simulink model "PMmotorFocECE517"  (R2018a)
settings: Solver=ode23t  StartTime=0  StopTime=0.1  FixedStep=1e-6  MaxStep=10e-7  RelTol=1e-8  EnableMultiTasking=on
InitFcn:
  | clc
  | clear
  | 
  | % DC Bus votlage
  | battery.Udc = 240;
  | 
  | % Motor
  | mtr.Ld = 400e-6;
  | mtr.Lq = 800e-6;
  | mtr.Rs = 0.05;
  | mtr.Lamda = 0.08;
  | mtr.Np = 3;
  | mtr.Jrotor = 0.03;
  | mtr.Tf = 3;
  | mtr.maxCurrLim = 280;
  | 
  | % inverter
  | Inv.RSnubber = 1e5;
  | Inv.Ron = 1e-3;
  | Inv.FrePWM = 10e3;
  | 
  | % current regulator
  | currCtrl.PI.wc = Inv.FrePWM/10*2*pi;
  | currCtrl.PI.Kpd = mtr.Ld*currCtrl.PI.wc;
  | currCtrl.PI.Kid = mtr.Rs*currCtrl.PI.wc;
  | currCtrl.PI.Kcd = 0.08;
  | currCtrl.PI.Kpq = mtr.Lq*currCtrl.PI.wc;
  | currCtrl.PI.Kiq = mtr.Rs*currCtrl.PI.wc;
  | currCtrl.PI.Kcq = 0.08;
  | currCtrl.voltageLim = battery.Udc*0.9;
  | 
  | % speed regulator
  | spdCtrl.PI.Kp = 12;
  | spdCtrl.PI.Ki= 3;
  | spdCtrl.PI.Kc  = 0.08;
  | 
  | %Field Weakening
  | fieldWeakening.PI.Kp = 0.3;
  | fieldWeakening.PI.Ki = 120;
  | fieldWeakening.PI.Kc = 3;
  | fieldWeakening.betaFLim = 90;  % deg
libraries: simulink x5, powerlib x5
settings Model: Creator=Rui Guan  LastModifiedBy=future
settings SolverCC: ZeroCrossControl=DisableAll  AlgebraicLoopSolver=LineSearch
settings DataIOCC: SaveFormat=Array  SignalLoggingSaveFormat=ModelDataLogs  SaveOutput=off  SignalLogging=off  DSMLogging=off  SaveTime=off
settings OptimizationCC: ExpressionDepthLimit=2147483647  LifeSpan=inf
settings DebuggingCC: UnderspecifiedInitializationDetection=Classic  MergeDetectMultiDrivingBlocksExec=none  SolverPrmCheckMsg=warning  FcnCallInpInsideContextMsg=warning  StateNameClashWarn=warning  SFUnexpectedBacktrackingDiag=warning  SFNoUnconditionalDefaultTransitionDiag=warning  SFExecutionAtInitializationDiag=none
settings HardwareCC: ProdBitPerPointer=32  ProdBitPerSizeT=32  ProdBitPerPtrDiffT=32  ProdLargestAtomicFloat=None  ProdIntDivRoundTo=Undefined  ProdEndianess=Unspecified  ProdWordSize=32  ProdHWDeviceType=32-bit Generic
settings ModelReferenceCC: PropagateSignalLabelsOutOfModel=off
settings CodeAppCC: StateflowObjectComments=on
settings GRTTargetCC: TargetLangStandard=C89/C90 (ANSI)  GeneratePreprocessorConditionals=Disable all  CombineOutputUpdateFcns=off  GRTInterface=on
settings ConfigComp: CovMetricSettings=dw  CovHtmlReporting=on  CovSaveCumulativeToWorkspaceVar=on  CovSaveSingleToWorkspaceVar=on  CovExternalEMLEnable=off
settings SimscapeCC: SimscapeNormalizeSystem=off

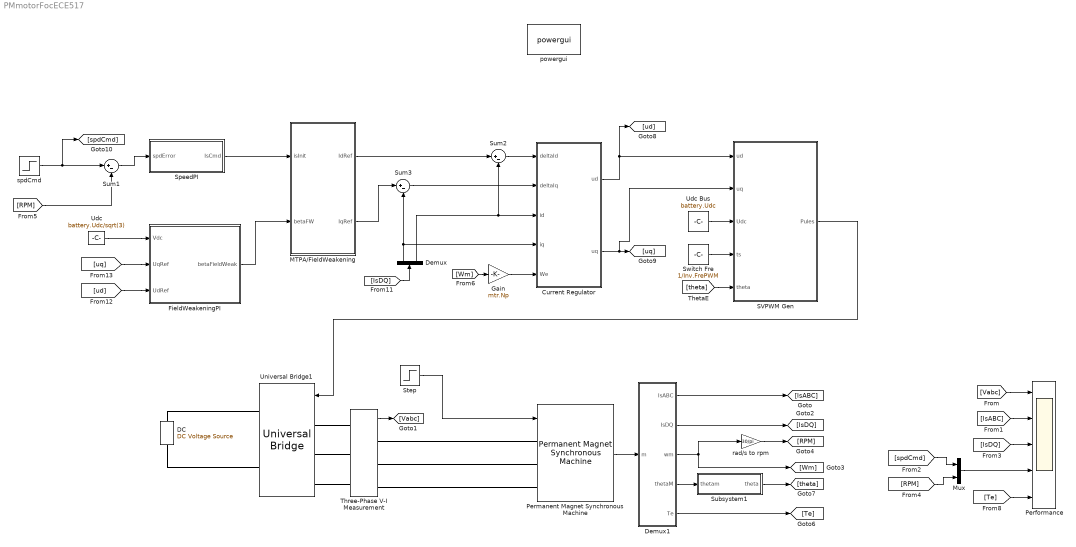
== system PMmotorFocECE517 ==
  " Udc Bus" : Constant  Value=battery.Udc
  " rad/s to rpm" : Gain  Gain=30/pi
  Current Regulator : Subsystem
  DC : powerlib/Electrical Sources/DC Voltage Source  Amplitude=battery.Udc  Measurements=Voltage
  Demux : Demux  Outputs=2
  Demux1 : Subsystem
  FieldWeakeningPI : Subsystem
  Gain : Gain  Gain=mtr.Np
  MTPA/FieldWeakening : Subsystem
  Mux : Mux  Inputs=2
  Performance : Scope  NumInputPorts=5
  Permanent Magnet Synchronous Machine : powerlib/Machines/Permanent Magnet Synchronous Machine  NbPhases=3  FluxDistribution=Sinusoidal  RotorType=Salient-pole  MechanicalLoad=Torque Tm  PresetModel=No  ShowDetailedParameters=on  MeasurementBus=off  Resistance=mtr.Rs  Inductance=8.5e-3  dqInductances=[mtr.Ld, mtr.Lq]  La=0.000835  MachineConstant=Flux linkage established by magnets (V.s)  Flux=mtr.Lamda  VoltageCst=43.5312  TorqueCst=0.36  Flat=120  Mechanical=[mtr.Jrotor 0 mtr.Tf]  PolePairs=3  InitialConditions=[0,0, 0,0]  InitialConditions5ph=[0 0 0 0 0 0]  TsPowergui=0  TsBlock=-1  RefAngle=90 degrees behind phase A axis (modified Park)
      settings: SourceProductName=Simscape Power Systems
  SVPWM Gen : Subsystem
  SpeedPI : Subsystem
  Step : Step  Time=0.2  Before=10  After=10  SampleTime=0
  Subsystem1 : Subsystem
  Sum1 : Sum  Inputs=|+-
  Sum2 : Sum  Inputs=|+-
  Sum3 : Sum  Inputs=|+-
  Switch Fre : Constant  Value=1/Inv.FrePWM  VectorParams1D=off
  Three-Phase V-I Measurement : powerlib/Measurements/Three-Phase V-I Measurement  VoltageMeasurement=phase-to-phase  SetLabelV=off  LabelV=Vabc  Vpu=off  VpuLL=off  CurrentMeasurement=no  SetLabelI=off  LabelI=Iabc  Ipu=off  Pbase=100e6  Vbase=500e3  OutputType=Complex  PhasorSimulation=off  PSBequivalent=0
  Udc : Constant  Value=battery.Udc/sqrt(3)
  Universal Bridge1 : powerlib/Power Electronics/Universal Bridge  Arms=3  SnubberResistance=Inv.RSnubber  SnubberCapacitance=inf  Device=IGBT / Diodes  Ron=Inv.Ron  Lon=0  ForwardVoltages="[  0  0  ]"  ForwardVoltage=0  GTOparameters=[ 10e-6 , 20e-6 ]  IGBTparameters=[ 1e-6 , 2e-6 ]  Measurements=None  Measurements_2=None  converterType=Rectifier
  powergui : powerlib/powergui  Priority=2  SimulationMode=Continuous  SampleTime=1e-6  frequency=60  Iterations=50  frequencyindice=0  Pbase=100e6  ErrMax=1e-4  UnitsV=kV  UnitsW=MW  buscounter=0  FunctionMessages=off  echomessages=off  EnableUseOfTLC=off  CurrentSourceSwitches=off  DisableSnubberDevices=off  DisableRonSwitches=off  DisableVfSwitches=off  DisplayEquations=off  SolverType=Tustin  Interpol=off  ExternalGateDelay=off  methode=off  Ts=0  x0status=blocks  SPID=off  SwTol=0  HookPort=off  RestoreLinks=warning  ResistiveCurrentMeasurement=off  Frange=[0:2:500]  Ylog=off  Xlog=on  ShowGrid=off  save=off  variable=ZData  structure=0  ZoomFFT=on  StartTime=0.0  cycles=1  DisplayStyle=1  fundamental=60  FreqAxis=off  MaxFrequency=1000  frequencyindicesteady=1  RmsSteady=1  display=off
  spdCmd : Step  Time=0.05  Before=1500  After=3000
  wires:
  Switch Fre/1 -> SVPWM Gen/4(ts)
  Permanent Magnet Synchronous Machine/1 -> Demux1/1(m)
  spdCmd/1 -> [spdCmd], Sum1/1
  Demux1/3(wm) -> " rad/s to rpm"/1, [Wm]
  Step/1 -> Permanent Magnet Synchronous Machine/1
  " Udc Bus"/1 -> SVPWM Gen/3(Udc)
  Sum2/1 -> Current Regulator/1(deltaId)
  Sum3/1 -> Current Regulator/2(deltaIq)
  MTPA/FieldWeakening/1(IdRef) -> Sum2/1
  MTPA/FieldWeakening/2(IqRef) -> Sum3/1
  SVPWM Gen/1(Pules) -> Universal Bridge1/1
  Three-Phase V-I Measurement/1 -> [Vabc]
  [Vabc] -> Performance/1
  Demux1/1(IsABC) -> [IsABC]
  [IsABC] -> Performance/2
  Demux1/2(IsDQ) -> [IsDQ]
  [IsDQ] -> Performance/3
  " rad/s to rpm"/1 -> [RPM]
  [RPM] -> Sum1/2
  [Wm] -> Gain/1
  Gain/1 -> Current Regulator/5(We)
  Demux1/4(thetaM) -> Subsystem1/1(thetam)
  Demux1/5(Te) -> [Te]
  [Te] -> Performance/5
  Subsystem1/1(theta) -> [theta]
  Demux/2 -> Sum2/2, Current Regulator/3(id)
  Demux/1 -> Sum3/2, Current Regulator/4(iq)
  [IsDQ] -> Demux/1
  Current Regulator/1(ud) -> [ud], SVPWM Gen/1(ud)
  Current Regulator/2(uq) -> SVPWM Gen/2(uq), [uq]
  FieldWeakeningPI/1(betaFieldWeak) -> MTPA/FieldWeakening/2(betaFW)
  Udc/1 -> FieldWeakeningPI/1(Vdc)
  [uq] -> FieldWeakeningPI/2(UqRef)
  [ud] -> FieldWeakeningPI/3(UdRef)
  Mux/1 -> Performance/4
  [RPM] -> Mux/2
  [spdCmd] -> Mux/1
  [theta] -> SVPWM Gen/5(theta)
  SpeedPI/1(IsCmd) -> MTPA/FieldWeakening/1(isInit)
  Sum1/1 -> SpeedPI/1(spdError)
  connections:
  DC/RConn1 -- Universal Bridge1/RConn1
  DC/LConn1 -- Universal Bridge1/RConn2
  Three-Phase V-I Measurement/LConn1 -- Universal Bridge1/LConn1
  Three-Phase V-I Measurement/LConn2 -- Universal Bridge1/LConn2
  Three-Phase V-I Measurement/LConn3 -- Universal Bridge1/LConn3
  Three-Phase V-I Measurement/RConn1 -- Permanent Magnet Synchronous Machine/LConn1
  Three-Phase V-I Measurement/RConn2 -- Permanent Magnet Synchronous Machine/LConn2
  Three-Phase V-I Measurement/RConn3 -- Permanent Magnet Synchronous Machine/LConn3

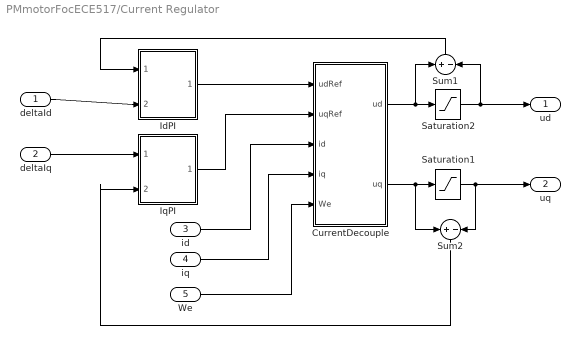
== system PMmotorFocECE517/Current Regulator ==
  deltaId : Inport
  deltaIq : Inport  Port=2
  id : Inport  Port=3
  iq : Inport  Port=4
  We : Inport  Port=5
  CurrentDecouple : Subsystem
  IdPI : Subsystem
  IqPI : Subsystem
  Saturation1 : Saturate  UpperLimit=currCtrl.voltageLim  LowerLimit=-currCtrl.voltageLim
  Saturation2 : Saturate  UpperLimit=currCtrl.voltageLim  LowerLimit=-currCtrl.voltageLim
  Sum1 : Sum  Inputs=+-  OutDataTypeStr=Inherit: Same as first input
  Sum2 : Sum  Inputs=+-  OutDataTypeStr=Inherit: Same as first input
  ud : Outport
  uq : Outport  Port=2
  wires:
  id/1 -> CurrentDecouple/3(id)
  CurrentDecouple/1(ud) -> Saturation2/1, Sum1/1
  iq/1 -> CurrentDecouple/4(iq)
  deltaIq/1 -> IqPI/1(iqError)
  IqPI/1(uqRef) -> CurrentDecouple/2(uqRef)
  We/1 -> CurrentDecouple/5(We)
  IdPI/1(udRef) -> CurrentDecouple/1(udRef)
  Saturation1/1 -> uq/1, Sum2/2
  CurrentDecouple/2(uq) -> Saturation1/1, Sum2/1
  Saturation2/1 -> ud/1, Sum1/2
  deltaId/1 -> IdPI/2(idError)
  Sum1/1 -> IdPI/1(udError)
  Sum2/1 -> IqPI/2(uqError)

== system PMmotorFocECE517/Demux1 ==
  m : Inport
  Bus Selector1 : BusSelector  OutputSignals=Stator current is_a (A),Stator current is_b (A),Stator current is_c (A),Stator current is_q (A),Stator current is_d (A),Rotor speed wm (rad/s),Rotor angle thetam (rad),Electromagnetic torque Te (N*m)
  Mux : Mux  Inputs=3
  Mux1 : Mux  Inputs=2
  IsABC : Outport
  IsDQ : Outport  Port=2
  wm : Outport  Port=3
  thetaM : Outport  Port=4
  Te : Outport  Port=5
  wires:
  m/1 -> Bus Selector1/1
  Bus Selector1/1 -> Mux/1  "<Stator current is_a (A)>"
  Bus Selector1/2 -> Mux/2  "<Stator current is_b (A)>"
  Bus Selector1/3 -> Mux/3  "<Stator current is_c (A)>"
  Bus Selector1/6 -> wm/1  "<Rotor speed wm (rad/s)>"
  Bus Selector1/7 -> thetaM/1  "<Rotor angle thetam (rad)>"
  Bus Selector1/8 -> Te/1  "<Electromagnetic torque Te (N*m)>"
  Mux/1 -> IsABC/1
  Bus Selector1/5 -> Mux1/2  "<Stator current is_d (A)>"
  Bus Selector1/4 -> Mux1/1  "<Stator current is_q (A)>"
  Mux1/1 -> IsDQ/1

== system PMmotorFocECE517/FieldWeakeningPI ==
  Vdc : Inport
  UqRef : Inport  Port=2
  UdRef : Inport  Port=3
  FieldWeakeningPICtrl : Subsystem
  Mux2 : Mux  Inputs=2
  Saturation : Saturate  UpperLimit=0  LowerLimit=-fieldWeakening.betaFLim
  Sum4 : Sum  Inputs=+-
  UMag : Fcn  Expr=sqrt(u[1]^2+u[2]^2)
  betaFieldWeak : Outport
  wires:
  UqRef/1 -> Mux2/1
  UdRef/1 -> Mux2/2
  Sum4/1 -> FieldWeakeningPICtrl/1(Error)
  Saturation/1 -> betaFieldWeak/1
  Vdc/1 -> Sum4/1
  UMag/1 -> Sum4/2
  Mux2/1 -> UMag/1
  FieldWeakeningPICtrl/1(Betaf) -> Saturation/1

== system PMmotorFocECE517/MTPA//FieldWeakening ==
  isInit : Inport
  betaFW : Inport  Port=2
  CurrentBetaToIdIq : Subsystem
  MTPA : Subsystem
  Sum5 : Sum  Inputs=+-
  IdRef : Outport
  IqRef : Outport  Port=2
  wires:
  MTPA/1(beta) -> Sum5/1
  isInit/1 -> MTPA/1(is), CurrentBetaToIdIq/2(is)
  betaFW/1 -> Sum5/2
  CurrentBetaToIdIq/1(id) -> IdRef/1
  CurrentBetaToIdIq/2(iq) -> IqRef/1
  Sum5/1 -> CurrentBetaToIdIq/1("beta ")

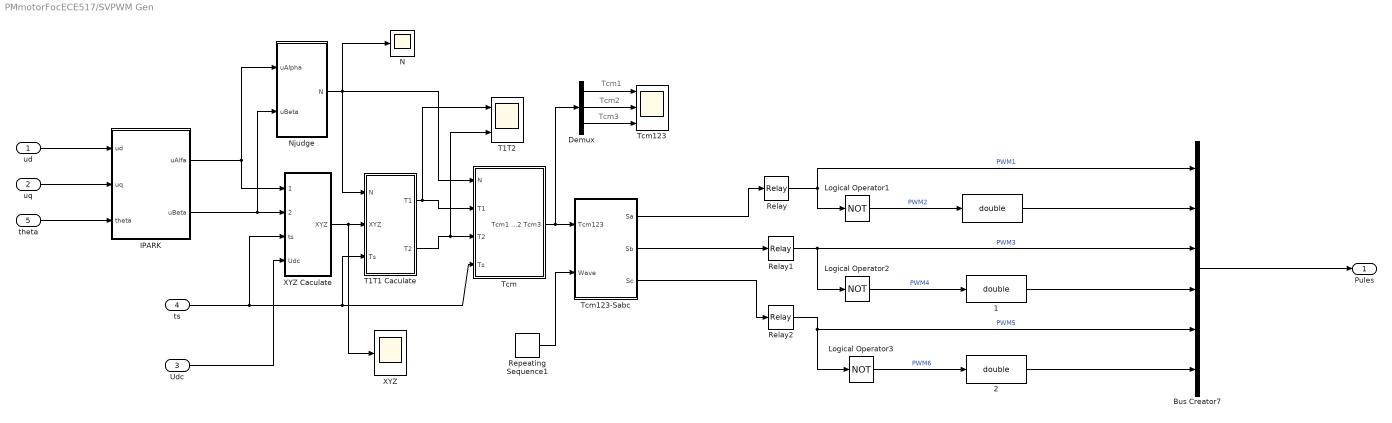
== system PMmotorFocECE517/SVPWM Gen ==
  note: Tcm1
  note: Tcm2
  note: Tcm3
  ud : Inport
  uq : Inport  Port=2
  Udc : Inport  Port=3
  ts : Inport  Port=4
  theta : Inport  Port=5
  "  " : DataTypeConversion  OutDataTypeStr=double
  "  1" : DataTypeConversion  OutDataTypeStr=double
  "  2" : DataTypeConversion  OutDataTypeStr=double
  Bus Creator7 : BusCreator  Inputs=6
  Demux : Demux  Outputs=3
  "IPARK " : Subsystem
  Logical Operator1 : Logic  Operator=NOT  AllPortsSameDT=off
  Logical Operator2 : Logic  Operator=NOT  AllPortsSameDT=off
  Logical Operator3 : Logic  Operator=NOT  AllPortsSameDT=off
  N : Scope
  Njudge : Subsystem
  Relay : Relay
  Relay1 : Relay
  Relay2 : Relay
  Repeating Sequence1 : simulink/Sources/Repeating Sequence  rep_seq_t="[0 1/2/Inv.FrePWM  1/Inv.FrePWM]"  rep_seq_y=[0 1/2/Inv.FrePWM 0]
  T1T1 Caculate : Subsystem  TreatAsAtomicUnit=on
  T1T2 : Scope  NumInputPorts=2
  Tcm : Subsystem
  Tcm123 : Scope  NumInputPorts=3
  Tcm123-Sabc : Subsystem
  XYZ : Scope
  "XYZ Caculate " : Subsystem
  Pules : Outport
  wires:
  "IPARK "/1(uAlfa) -> "XYZ Caculate "/1(uAlpha), Njudge/1(uAlpha)
  "XYZ Caculate "/1(XYZ) -> XYZ/1, T1T1 Caculate/2(XYZ)
  T1T1 Caculate/1(T1) -> T1T2/1, Tcm/2(T1)
  T1T1 Caculate/2(T2) -> T1T2/2, Tcm/3(T2)
  Njudge/1("N ") -> N/1, T1T1 Caculate/1(N), Tcm/1(N)
  Tcm/1(Tcm1 Tcm2 Tcm3) -> Demux/1, Tcm123-Sabc/1(Tcm123)
  Repeating Sequence1/1 -> Tcm123-Sabc/2(Wave)
  Demux/1 -> Tcm123/1
  Demux/2 -> Tcm123/2
  Demux/3 -> Tcm123/3
  Udc/1 -> "XYZ Caculate "/4(Udc)
  ts/1 -> "XYZ Caculate "/3(ts), T1T1 Caculate/3(Ts), Tcm/4(Ts)
  "IPARK "/2(uBeta) -> "XYZ Caculate "/2(uBeta), Njudge/2(uBeta)
  "  2"/1 -> Bus Creator7/6
  Logical Operator3/1 -> "  2"/1  "PWM6"
  "  1"/1 -> Bus Creator7/4
  Logical Operator2/1 -> "  1"/1  "PWM4"
  Logical Operator1/1 -> "  "/1  "PWM2"
  "  "/1 -> Bus Creator7/2
  Bus Creator7/1 -> Pules/1
  Relay2/1 -> Bus Creator7/5, Logical Operator3/1  "PWM5"
  Relay1/1 -> Bus Creator7/3, Logical Operator2/1  "PWM3"
  Relay/1 -> Bus Creator7/1, Logical Operator1/1  "PWM1"
  Tcm123-Sabc/3(Sc) -> Relay2/1
  Tcm123-Sabc/2(Sb) -> Relay1/1
  Tcm123-Sabc/1(Sa) -> Relay/1
  ud/1 -> "IPARK "/1(ud)
  uq/1 -> "IPARK "/2(uq)
  theta/1 -> "IPARK "/3(theta)

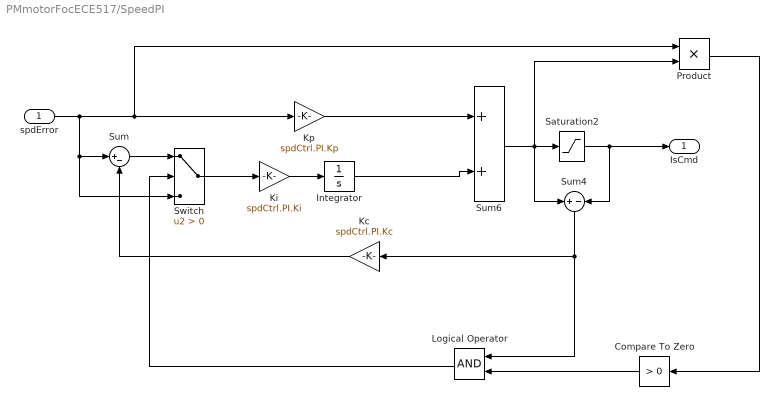
== system PMmotorFocECE517/SpeedPI ==
  spdError : Inport
  Compare To Zero : simulink/Logic and Bit Operations/Compare To Zero  relop=>  OutDataTypeStr=uint8  ZeroCross=off
  Integrator : Integrator
  Kc : Gain  Gain=spdCtrl.PI.Kc  OutDataTypeStr=Inherit: Same as input  ParamDataTypeStr=Inherit: Same as input
  Ki : Gain  Gain=spdCtrl.PI.Ki  OutDataTypeStr=Inherit: Same as input  ParamDataTypeStr=Inherit: Same as input
  Kp : Gain  Gain=spdCtrl.PI.Kp  OutDataTypeStr=Inherit: Same as input  ParamDataTypeStr=Inherit: Same as input
  Logical Operator : Logic  AllPortsSameDT=off  OutDataTypeStr=boolean
  Product : Product  RndMeth=Zero
  Saturation2 : Saturate  UpperLimit=mtr.maxCurrLim  LowerLimit=-mtr.maxCurrLim
  Sum : Sum  Inputs=|+-  OutDataTypeStr=Inherit: Same as first input
  Sum4 : Sum  Inputs=+-  OutDataTypeStr=Inherit: Same as first input
  Sum6 : Sum  SaturateOnIntegerOverflow=on  InputSameDT=on  OutDataTypeStr=Inherit: Same as first input
  Switch : Switch  Criteria=u2 > Threshold
  IsCmd : Outport
  wires:
  Compare To Zero/1 -> Logical Operator/2
  Sum4/1 -> Logical Operator/1, Kc/1
  Sum6/1 -> Saturation2/1, Sum4/1, Product/2
  Sum/1 -> Switch/1
  Product/1 -> Compare To Zero/1
  Logical Operator/1 -> Switch/2
  Switch/1 -> Ki/1
  Ki/1 -> Integrator/1
  Integrator/1 -> Sum6/2
  Saturation2/1 -> IsCmd/1, Sum4/2
  Kc/1 -> Sum/2
  Kp/1 -> Sum6/1
  spdError/1 -> Kp/1, Product/1, Sum/1, Switch/3

== system PMmotorFocECE517/Subsystem1 ==
  thetam : Inport
  Add1 : Sum  Inputs=+-
  Constant4 : Constant  Value=0.5*pi
  Gain1 : Gain  Gain=mtr.Np
  theta : Outport
  wires:
  Gain1/1 -> Add1/1
  Constant4/1 -> Add1/2
  Add1/1 -> theta/1
  thetam/1 -> Gain1/1

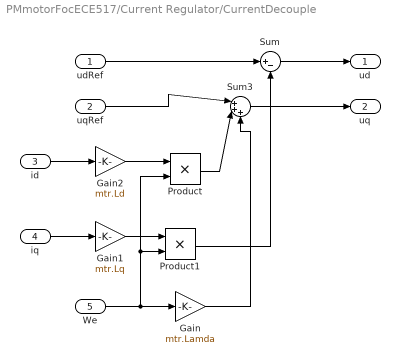
== system PMmotorFocECE517/Current Regulator/CurrentDecouple ==
  udRef : Inport
  uqRef : Inport  Port=2
  id : Inport  Port=3
  iq : Inport  Port=4
  We : Inport  Port=5
  Gain : Gain  Gain=mtr.Lamda
  Gain1 : Gain  Gain=mtr.Lq
  Gain2 : Gain  Gain=mtr.Ld
  Product : Product  RndMeth=Zero
  Product1 : Product  RndMeth=Zero
  Sum : Sum  Inputs=|+-
  Sum3 : Sum  Inputs=|+++
  ud : Outport
  uq : Outport  Port=2
  wires:
  Sum3/1 -> uq/1
  Product/1 -> Sum3/2
  uqRef/1 -> Sum3/1
  Gain/1 -> Sum3/3
  We/1 -> Product/2, Product1/2, Gain/1
  iq/1 -> Gain1/1
  udRef/1 -> Sum/1
  Product1/1 -> Sum/2
  Sum/1 -> ud/1
  Gain1/1 -> Product1/1
  Gain2/1 -> Product/1
  id/1 -> Gain2/1

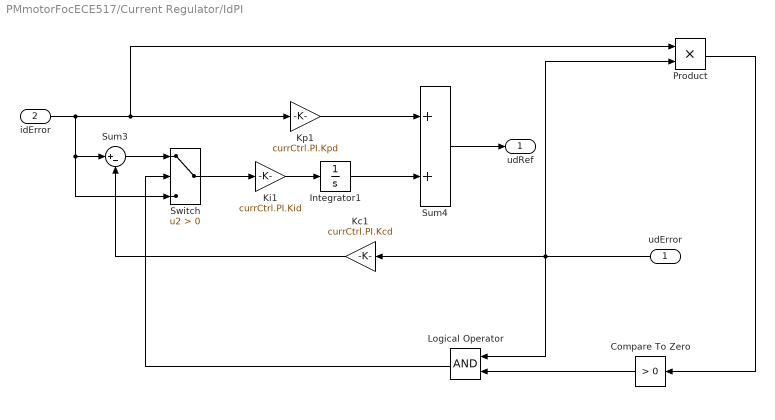
== system PMmotorFocECE517/Current Regulator/IdPI ==
  udError : Inport
  idError : Inport  Port=2
  Compare To Zero : simulink/Logic and Bit Operations/Compare To Zero  relop=>  OutDataTypeStr=uint8  ZeroCross=off
  Integrator1 : Integrator
  Kc1 : Gain  Gain=currCtrl.PI.Kcd  OutDataTypeStr=Inherit: Same as input  ParamDataTypeStr=Inherit: Same as input
  Ki1 : Gain  Gain=currCtrl.PI.Kid  OutDataTypeStr=Inherit: Same as input  ParamDataTypeStr=Inherit: Same as input
  Kp1 : Gain  Gain=currCtrl.PI.Kpd  OutDataTypeStr=Inherit: Same as input  ParamDataTypeStr=Inherit: Same as input
  Logical Operator : Logic  AllPortsSameDT=off  OutDataTypeStr=boolean
  Product : Product  RndMeth=Zero
  Sum3 : Sum  Inputs=|+-  OutDataTypeStr=Inherit: Same as first input
  Sum4 : Sum  SaturateOnIntegerOverflow=on  InputSameDT=on  OutDataTypeStr=Inherit: Same as first input
  Switch : Switch  Criteria=u2 > Threshold
  udRef : Outport
  wires:
  Switch/1 -> Ki1/1
  Ki1/1 -> Integrator1/1
  Sum4/1 -> udRef/1
  udError/1 -> Kc1/1, Product/2, Logical Operator/1
  Integrator1/1 -> Sum4/2
  Sum3/1 -> Switch/1
  Kc1/1 -> Sum3/2
  Kp1/1 -> Sum4/1
  Compare To Zero/1 -> Logical Operator/2
  Logical Operator/1 -> Switch/2
  idError/1 -> Kp1/1, Product/1, Sum3/1, Switch/3
  Product/1 -> Compare To Zero/1

== system PMmotorFocECE517/Current Regulator/IqPI ==
  iqError : Inport
  uqError : Inport  Port=2
  Compare To Zero : simulink/Logic and Bit Operations/Compare To Zero  relop=>  OutDataTypeStr=uint8  ZeroCross=off
  Integrator1 : Integrator
  Kc1 : Gain  Gain=currCtrl.PI.Kcq  OutDataTypeStr=Inherit: Same as input  ParamDataTypeStr=Inherit: Same as input
  Ki1 : Gain  Gain=currCtrl.PI.Kiq  OutDataTypeStr=Inherit: Same as input  ParamDataTypeStr=Inherit: Same as input
  Kp1 : Gain  Gain=currCtrl.PI.Kpq  OutDataTypeStr=Inherit: Same as input  ParamDataTypeStr=Inherit: Same as input
  Logical Operator : Logic  AllPortsSameDT=off  OutDataTypeStr=boolean
  Product : Product  RndMeth=Zero
  Sum3 : Sum  Inputs=|+-  OutDataTypeStr=Inherit: Same as first input
  Sum4 : Sum  SaturateOnIntegerOverflow=on  InputSameDT=on  OutDataTypeStr=Inherit: Same as first input
  Switch : Switch  Criteria=u2 > Threshold
  uqRef : Outport
  wires:
  Ki1/1 -> Integrator1/1
  Integrator1/1 -> Sum4/2
  Product/1 -> Compare To Zero/1
  Switch/1 -> Ki1/1
  iqError/1 -> Kp1/1, Product/1, Sum3/1, Switch/3
  Compare To Zero/1 -> Logical Operator/2
  Logical Operator/1 -> Switch/2
  Kp1/1 -> Sum4/1
  Sum3/1 -> Switch/1
  Sum4/1 -> uqRef/1
  uqError/1 -> Kc1/1, Product/2, Logical Operator/1
  Kc1/1 -> Sum3/2

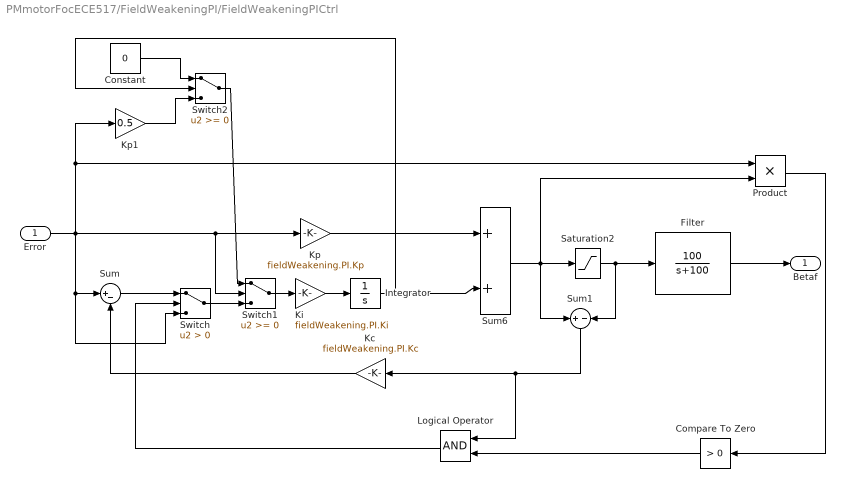
== system PMmotorFocECE517/FieldWeakeningPI/FieldWeakeningPICtrl ==
  Error : Inport
  Compare To Zero : simulink/Logic and Bit Operations/Compare To Zero  relop=>  OutDataTypeStr=uint8  ZeroCross=off
  Constant : Constant  Value=0
  Filter : TransferFcn  Numerator=[100]  Denominator=[1 100]
  Integrator : Integrator
  Kc : Gain  Gain=fieldWeakening.PI.Kc  OutDataTypeStr=Inherit: Same as input  ParamDataTypeStr=Inherit: Same as input
  Ki : Gain  Gain=fieldWeakening.PI.Ki  OutDataTypeStr=Inherit: Same as input  ParamDataTypeStr=Inherit: Same as input
  Kp : Gain  Gain=fieldWeakening.PI.Kp  OutDataTypeStr=Inherit: Same as input  ParamDataTypeStr=Inherit: Same as input
  Kp1 : Gain  Gain=0.5  OutDataTypeStr=Inherit: Same as input  ParamDataTypeStr=Inherit: Same as input
  Logical Operator : Logic  AllPortsSameDT=off  OutDataTypeStr=boolean
  Product : Product  RndMeth=Zero
  Saturation2 : Saturate  UpperLimit=fieldWeakening.betaFLim  LowerLimit=-fieldWeakening.betaFLim
  Sum : Sum  Inputs=|+-  OutDataTypeStr=Inherit: Same as first input
  Sum1 : Sum  Inputs=+-  OutDataTypeStr=Inherit: Same as first input
  Sum6 : Sum  SaturateOnIntegerOverflow=on  InputSameDT=on  OutDataTypeStr=Inherit: Same as first input
  Switch : Switch  Criteria=u2 > Threshold
  Switch1 : Switch
  Switch2 : Switch
  Betaf : Outport
  wires:
  Kp/1 -> Sum6/1
  Switch1/1 -> Ki/1
  Kp1/1 -> Switch2/3
  Kc/1 -> Sum/2
  Constant/1 -> Switch2/1
  Product/1 -> Compare To Zero/1
  Sum1/1 -> Kc/1, Logical Operator/1
  Error/1 -> Kp/1, Switch1/2, Product/1, Kp1/1, Sum/1, Switch/3
  Switch/1 -> Switch1/3
  Ki/1 -> Integrator/1
  Integrator/1 -> Sum6/2, Switch2/2
  Sum/1 -> Switch/1
  Compare To Zero/1 -> Logical Operator/2
  Switch2/1 -> Switch1/1
  Logical Operator/1 -> Switch/2
  Filter/1 -> Betaf/1
  Sum6/1 -> Product/2, Sum1/1, Saturation2/1
  Saturation2/1 -> Filter/1, Sum1/2

== system PMmotorFocECE517/MTPA//FieldWeakening/CurrentBetaToIdIq ==
  "beta " : Inport
  is : Inport  Port=2
  Gain1 : Gain  Gain=pi/180
  Product : Product  RndMeth=Zero
  Product1 : Product  RndMeth=Zero
  Trigonometric Function : Trigonometry
  Trigonometric Function1 : Trigonometry  Operator=cos
  id : Outport
  iq : Outport  Port=2
  wires:
  Product/1 -> iq/1
  Product1/1 -> id/1
  Trigonometric Function/1 -> Product/1
  "beta "/1 -> Gain1/1
  is/1 -> Product1/1, Product/2
  Gain1/1 -> Trigonometric Function/1, Trigonometric Function1/1
  Trigonometric Function1/1 -> Product1/2

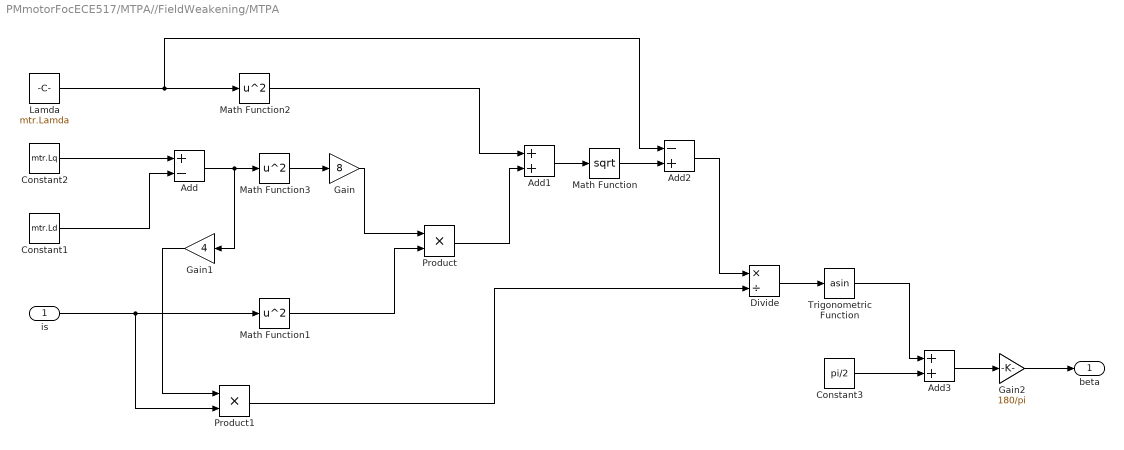
== system PMmotorFocECE517/MTPA//FieldWeakening/MTPA ==
  is : Inport
  Add : Sum  Inputs=+-
  Add1 : Sum
  Add2 : Sum  Inputs=-+
  Add3 : Sum
  Constant1 : Constant  Value=mtr.Ld
  Constant2 : Constant  Value=mtr.Lq
  Constant3 : Constant  Value=pi/2
  Divide : Product  Inputs=*/
  Gain : Gain  Gain=8
  Gain1 : Gain  Gain=4
  Gain2 : Gain  Gain=180/pi
  Lamda : Constant  Value=mtr.Lamda
  Math Function : Math  Operator=sqrt  SaturateOnIntegerOverflow=on
  Math Function1 : Math  Operator=square  SaturateOnIntegerOverflow=on
  Math Function2 : Math  Operator=square  SaturateOnIntegerOverflow=on
  Math Function3 : Math  Operator=square  SaturateOnIntegerOverflow=on
  Product : Product  RndMeth=Zero
  Product1 : Product  RndMeth=Zero
  Trigonometric Function : Trigonometry  Operator=asin
  beta : Outport
  wires:
  Divide/1 -> Trigonometric Function/1
  Add1/1 -> Math Function/1
  Math Function/1 -> Add2/2
  Gain2/1 -> beta/1
  Constant1/1 -> Add/2
  Trigonometric Function/1 -> Add3/1
  is/1 -> Product1/2, Math Function1/1
  Add3/1 -> Gain2/1
  Add/1 -> Math Function3/1, Gain1/1
  Gain/1 -> Product/1
  Math Function2/1 -> Add1/1
  Gain1/1 -> Product1/1
  Product/1 -> Add1/2
  Product1/1 -> Divide/2
  Math Function3/1 -> Gain/1
  Math Function1/1 -> Product/2
  Lamda/1 -> Math Function2/1, Add2/1
  Add2/1 -> Divide/1
  Constant2/1 -> Add/1
  Constant3/1 -> Add3/2

== system PMmotorFocECE517/SVPWM Gen/IPARK  ==
  ud : Inport
  uq : Inport  Port=2
  theta : Inport  Port=3
  Mux : Mux  Inputs=3
  uAlfaFuc : Fcn  Expr=u(1)*cos(u(3))-u(2)*sin(u(3))
  uBetaFuc : Fcn  Expr=u(1)*sin(u(3))+u(2)*cos(u(3))
  uAlfa : Outport
  uBeta : Outport  Port=2
  wires:
  uBetaFuc/1 -> uBeta/1
  theta/1 -> Mux/3
  uq/1 -> Mux/2
  ud/1 -> Mux/1
  uAlfaFuc/1 -> uAlfa/1
  Mux/1 -> uBetaFuc/1, uAlfaFuc/1

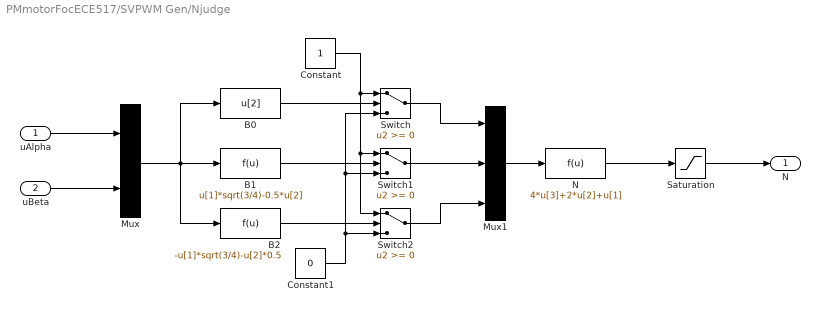
== system PMmotorFocECE517/SVPWM Gen/Njudge ==
  uAlpha : Inport
  uBeta : Inport  Port=2
  B0 : Fcn  Expr=u[2]
  B1 : Fcn  Expr=u[1]*sqrt(3/4)-0.5*u[2]
  B2 : Fcn  Expr=-u[1]*sqrt(3/4)-u[2]*0.5
  Constant : Constant
  Constant1 : Constant  Value=0
  Mux : Mux  Inputs=2
  Mux1 : Mux  Inputs=3
  N : Fcn  Expr=4*u[3]+2*u[2]+u[1]
  Saturation : Saturate  UpperLimit=6  LowerLimit=1
  Switch : Switch
  Switch1 : Switch
  Switch2 : Switch
  "N " : Outport
  wires:
  N/1 -> Saturation/1
  Mux1/1 -> N/1
  Switch1/1 -> Mux1/2
  Constant1/1 -> Switch2/3, Switch1/3, Switch/3
  Constant/1 -> Switch1/1, Switch2/1, Switch/1
  B2/1 -> Switch2/2
  B1/1 -> Switch1/2
  B0/1 -> Switch/2
  Mux/1 -> B2/1, B0/1, B1/1
  uBeta/1 -> Mux/2
  uAlpha/1 -> Mux/1
  Switch/1 -> Mux1/1
  Switch2/1 -> Mux1/3
  Saturation/1 -> "N "/1

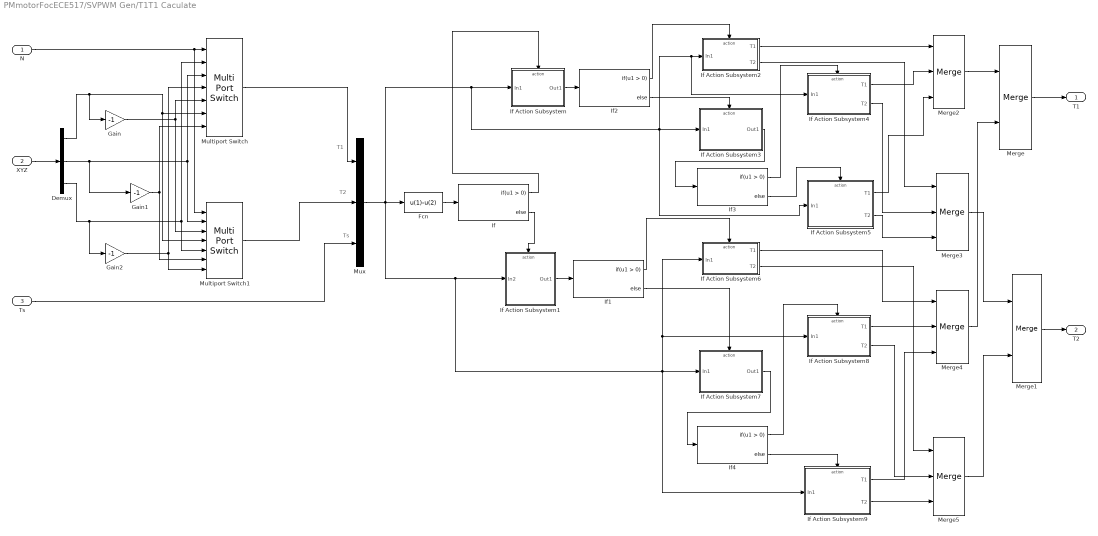
== system PMmotorFocECE517/SVPWM Gen/T1T1 Caculate ==
  note: Ts
  note: T2
  note: T1
  N : Inport
  XYZ : Inport  Port=2
  Ts : Inport  Port=3
  Demux : Demux  Outputs=3
  Fcn : Fcn  Expr=u(1)-u(2)
  Gain : Gain  Gain=-1  OutDataTypeStr=Inherit: Same as input  ParamDataTypeStr=Inherit: Same as input
  Gain1 : Gain  Gain=-1  OutDataTypeStr=Inherit: Same as input  ParamDataTypeStr=Inherit: Same as input
  Gain2 : Gain  Gain=-1  OutDataTypeStr=Inherit: Same as input  ParamDataTypeStr=Inherit: Same as input
  If{,1..4} (5 alike) : If
  If Action Subsystem : Subsystem  TreatAsAtomicUnit=on
  If Action Subsystem1 : Subsystem  TreatAsAtomicUnit=on
  If Action Subsystem2 : Subsystem  TreatAsAtomicUnit=on
  If Action Subsystem3 : Subsystem  TreatAsAtomicUnit=on
  If Action Subsystem4 : Subsystem  TreatAsAtomicUnit=on
  If Action Subsystem5 : Subsystem  TreatAsAtomicUnit=on
  If Action Subsystem6 : Subsystem  TreatAsAtomicUnit=on
  If Action Subsystem7 : Subsystem  TreatAsAtomicUnit=on
  If Action Subsystem8 : Subsystem  TreatAsAtomicUnit=on
  If Action Subsystem9 : Subsystem  TreatAsAtomicUnit=on
  Merge : Merge
  Merge1 : Merge
  Merge{2..5} (4 alike) : Merge  Inputs=3
  Multiport Switch : MultiPortSwitch  Inputs=6
  Multiport Switch1 : MultiPortSwitch  Inputs=6
  Mux : Mux  Inputs=3
  T1 : Outport
  T2 : Outport  Port=2
  wires:
  If4/2 -> If Action Subsystem9/Action
  If4/1 -> If Action Subsystem8/Action
  If Action Subsystem7/1(Out1) -> If4/1
  If3/2 -> If Action Subsystem5/Action
  If3/1 -> If Action Subsystem4/Action
  If Action Subsystem3/1(Out1) -> If3/1
  If1/1 -> If Action Subsystem6/Action
  If Action Subsystem1/1(Out1) -> If1/1
  If2/2 -> If Action Subsystem3/Action
  If2/1 -> If Action Subsystem2/Action
  If Action Subsystem/1(Out1) -> If2/1
  Gain1/1 -> Multiport Switch/7, Multiport Switch1/6
  Gain2/1 -> Multiport Switch1/7, Multiport Switch/4
  Gain/1 -> Multiport Switch/5, Multiport Switch1/3
  Demux/1 -> Gain/1, Multiport Switch1/4, Multiport Switch/6
  Demux/3 -> Gain2/1, Multiport Switch/2, Multiport Switch1/5
  Demux/2 -> Gain1/1, Multiport Switch1/2, Multiport Switch/3
  Multiport Switch1/1 -> Mux/2
  Multiport Switch/1 -> Mux/1
  Mux/1 -> If Action Subsystem9/1(In1), If Action Subsystem8/1(In1), If Action Subsystem6/1(In1), If Action Subsystem7/1(In1), If Action Subsystem1/1(In2), If Action Subsystem/1(In1), If Action Subsystem5/1(In1), If Action Subsystem4/1(In1), If Action Subsystem2/1(In1), If Action Subsystem3/1(In1), Fcn/1
  XYZ/1 -> Demux/1
  Ts/1 -> Mux/3
  Fcn/1 -> If/1
  If/1 -> If Action Subsystem/Action
  If/2 -> If Action Subsystem1/Action
  Merge/1 -> T1/1
  Merge1/1 -> T2/1
  If Action Subsystem8/1(T1) -> Merge4/2
  If1/2 -> If Action Subsystem7/Action
  If Action Subsystem2/1(T1) -> Merge2/1
  If Action Subsystem4/1(T1) -> Merge2/2
  If Action Subsystem5/1(T1) -> Merge2/3
  If Action Subsystem2/2(T2) -> Merge3/1
  If Action Subsystem4/2(T2) -> Merge3/2
  If Action Subsystem5/2(T2) -> Merge3/3
  Merge2/1 -> Merge/1
  Merge3/1 -> Merge1/1
  Merge4/1 -> Merge/2
  Merge5/1 -> Merge1/2
  If Action Subsystem6/1(T1) -> Merge4/1
  If Action Subsystem9/1(T1) -> Merge4/3
  If Action Subsystem6/2(T2) -> Merge5/1
  If Action Subsystem8/2(T2) -> Merge5/2
  If Action Subsystem9/2(T2) -> Merge5/3
  N/1 -> Multiport Switch1/1, Multiport Switch/1

== system PMmotorFocECE517/SVPWM Gen/Tcm ==
  N : Inport
  T1 : Inport  Port=2
  T2 : Inport  Port=3
  Ts : Inport  Port=4
  Fcn : Fcn  Expr=(u[3]-u[1]-u[2])/4
  Fcn1 : Fcn  Expr=(u[3]+u[1]-u[2])/4
  Fcn2 : Fcn  Expr=(u[3]+u[2]+u[1])/4
  Multiport Switch : MultiPortSwitch  Inputs=6
  Multiport Switch1 : MultiPortSwitch  Inputs=6
  Multiport Switch2 : MultiPortSwitch  Inputs=6
  Mux : Mux  Inputs=3
  Mux1 : Mux  Inputs=3
  Tcm1 Tcm2 Tcm3 : Outport
  wires:
  N/1 -> Multiport Switch2/1, Multiport Switch1/1, Multiport Switch/1
  Fcn2/1 -> Multiport Switch2/4, Multiport Switch2/2, Multiport Switch1/7, Multiport Switch1/3, Multiport Switch/6, Multiport Switch/5
  Fcn1/1 -> Multiport Switch2/6, Multiport Switch2/3, Multiport Switch1/5, Multiport Switch1/4, Multiport Switch/2, Multiport Switch/7
  Fcn/1 -> Multiport Switch2/7, Multiport Switch2/5, Multiport Switch1/6, Multiport Switch1/2, Multiport Switch/4, Multiport Switch/3
  Mux1/1 -> Tcm1 Tcm2 Tcm3/1
  Multiport Switch/1 -> Mux1/1
  Multiport Switch1/1 -> Mux1/2
  Multiport Switch2/1 -> Mux1/3
  T1/1 -> Mux/1
  T2/1 -> Mux/2
  Ts/1 -> Mux/3
  Mux/1 -> Fcn1/1, Fcn/1, Fcn2/1

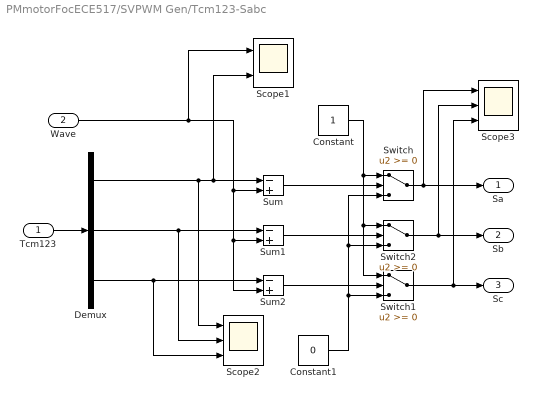
== system PMmotorFocECE517/SVPWM Gen/Tcm123-Sabc ==
  Tcm123 : Inport
  Wave : Inport  Port=2
  Constant : Constant
  Constant1 : Constant  Value=0
  Demux : Demux  Outputs=3
  Scope1 : Scope  NumInputPorts=2
  Scope2 : Scope  NumInputPorts=3
  Scope3 : Scope  NumInputPorts=3
  Sum : Sum  Inputs=-+  SaturateOnIntegerOverflow=on  OutDataTypeStr=Inherit: Same as first input
  Sum1 : Sum  Inputs=-+  SaturateOnIntegerOverflow=on  OutDataTypeStr=Inherit: Same as first input
  Sum2 : Sum  Inputs=-+  SaturateOnIntegerOverflow=on  OutDataTypeStr=Inherit: Same as first input
  Switch : Switch  SaturateOnIntegerOverflow=on
  Switch1 : Switch  SaturateOnIntegerOverflow=on
  Switch2 : Switch  SaturateOnIntegerOverflow=on
  Sa : Outport
  Sb : Outport  Port=2
  Sc : Outport  Port=3
  wires:
  Wave/1 -> Scope1/1, Sum/2, Sum2/2, Sum1/2
  Demux/1 -> Scope2/1, Sum/1, Scope1/2
  Demux/2 -> Scope2/2, Sum1/1
  Demux/3 -> Scope2/3, Sum2/1
  Tcm123/1 -> Demux/1
  Sum/1 -> Switch/2
  Sum1/1 -> Switch2/2
  Sum2/1 -> Switch1/2
  Constant/1 -> Switch1/1, Switch2/1, Switch/1
  Constant1/1 -> Switch/3, Switch2/3, Switch1/3
  Switch/1 -> Scope3/1, Sa/1
  Switch2/1 -> Scope3/2, Sb/1
  Switch1/1 -> Scope3/3, Sc/1

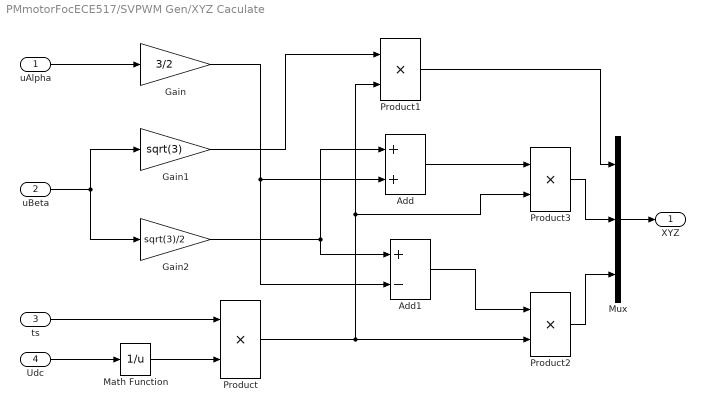
== system PMmotorFocECE517/SVPWM Gen/XYZ Caculate  ==
  uAlpha : Inport
  uBeta : Inport  Port=2
  ts : Inport  Port=3
  Udc : Inport  Port=4
  Add : Sum  OutDataTypeStr=Inherit: Same as first input
  Add1 : Sum  Inputs=+-  OutDataTypeStr=Inherit: Same as first input
  Gain : Gain  Gain=3/2  OutDataTypeStr=Inherit: Same as input  ParamDataTypeStr=Inherit: Same as input
  Gain1 : Gain  Gain=sqrt(3)  OutDataTypeStr=Inherit: Same as input  ParamDataTypeStr=Inherit: Same as input
  Gain2 : Gain  Gain=sqrt(3)/2  OutDataTypeStr=Inherit: Same as input  ParamDataTypeStr=Inherit: Same as input
  Math Function : Math  Operator=reciprocal  SaturateOnIntegerOverflow=on
  Mux : Mux  Inputs=3
  Product{,1..3} (4 alike) : Product  RndMeth=Zero  OutDataTypeStr=Inherit: Same as first input
  XYZ : Outport
  wires:
  Add/1 -> Product3/1
  Add1/1 -> Product2/1
  Gain2/1 -> Add1/1, Add/1
  Gain/1 -> Add/2, Add1/2
  Product/1 -> Product3/2, Product1/2, Product2/2
  Gain1/1 -> Product1/1
  ts/1 -> Product/1
  Math Function/1 -> Product/2
  Udc/1 -> Math Function/1
  uBeta/1 -> Gain1/1, Gain2/1
  uAlpha/1 -> Gain/1
  Product2/1 -> Mux/3
  Product3/1 -> Mux/2
  Product1/1 -> Mux/1
  Mux/1 -> XYZ/1

== system PMmotorFocECE517/SVPWM Gen/T1T1 Caculate/If Action Subsystem ==
  In1 : Inport
  Action Port : ActionPort  ActionType=then
  Fcn2 : Fcn  Expr=u(1)+u(2)/2-u(3)
  Out1 : Outport
  wires:
  Fcn2/1 -> Out1/1
  In1/1 -> Fcn2/1

== system PMmotorFocECE517/SVPWM Gen/T1T1 Caculate/If Action Subsystem1 ==
  In2 : Inport
  Action Port : ActionPort  ActionType=else
  Fcn1 : Fcn  Expr=u(2)+u(1)/2-u(3)
  Out1 : Outport
  wires:
  Fcn1/1 -> Out1/1
  In2/1 -> Fcn1/1

== system PMmotorFocECE517/SVPWM Gen/T1T1 Caculate/If Action Subsystem2 ==
  In1 : Inport
  Action Port : ActionPort  ActionType=then
  Fcn1 : Fcn  Expr=0
  T : Fcn  Expr=u(3)
  T1 : Outport
  T2 : Outport  Port=2
  wires:
  In1/1 -> T/1, Fcn1/1
  T/1 -> T1/1
  Fcn1/1 -> T2/1

== system PMmotorFocECE517/SVPWM Gen/T1T1 Caculate/If Action Subsystem3 ==
  In1 : Inport
  Action Port : ActionPort  ActionType=else
  Fcn : Fcn  Expr=u(1)+u(2)-u(3)
  Out1 : Outport
  wires:
  In1/1 -> Fcn/1
  Fcn/1 -> Out1/1

== system PMmotorFocECE517/SVPWM Gen/T1T1 Caculate/If Action Subsystem4 ==
  In1 : Inport
  Action Port : ActionPort  ActionType=then
  Fcn1 : Fcn  Expr=u(1)/(u(1)+u(2))*u(3)
  Fcn2 : Fcn  Expr=u(2)/(u(1)+u(2))*u(3)
  T1 : Outport
  T2 : Outport  Port=2
  wires:
  Fcn2/1 -> T2/1
  Fcn1/1 -> T1/1
  In1/1 -> Fcn2/1, Fcn1/1

== system PMmotorFocECE517/SVPWM Gen/T1T1 Caculate/If Action Subsystem5 ==
  In1 : Inport
  Action Port : ActionPort  ActionType=else
  Fcn1 : Fcn  Expr=u(1)
  Fcn2 : Fcn  Expr=u(2)
  T1 : Outport
  T2 : Outport  Port=2
  wires:
  In1/1 -> Fcn1/1, Fcn2/1
  Fcn1/1 -> T1/1
  Fcn2/1 -> T2/1

== system PMmotorFocECE517/SVPWM Gen/T1T1 Caculate/If Action Subsystem6 ==
  In1 : Inport
  Action Port : ActionPort  ActionType=then
  Fcn1 : Fcn  Expr=u(3)
  T : Fcn  Expr=0
  T1 : Outport
  T2 : Outport  Port=2
  wires:
  Fcn1/1 -> T2/1
  T/1 -> T1/1
  In1/1 -> Fcn1/1, T/1

== system PMmotorFocECE517/SVPWM Gen/T1T1 Caculate/If Action Subsystem7 ==
  In1 : Inport
  Action Port : ActionPort  ActionType=else
  Fcn : Fcn  Expr=u(1)+u(2)-u(3)
  Out1 : Outport
  wires:
  Fcn/1 -> Out1/1
  In1/1 -> Fcn/1

== system PMmotorFocECE517/SVPWM Gen/T1T1 Caculate/If Action Subsystem8 ==
  In1 : Inport
  Action Port : ActionPort  ActionType=then
  Fcn1 : Fcn  Expr=u(1)/(u(1)+u(2))*u(3)
  Fcn2 : Fcn  Expr=u(2)/(u(1)+u(2))*u(3)
  T1 : Outport
  T2 : Outport  Port=2
  wires:
  In1/1 -> Fcn1/1, Fcn2/1
  Fcn1/1 -> T1/1
  Fcn2/1 -> T2/1

== system PMmotorFocECE517/SVPWM Gen/T1T1 Caculate/If Action Subsystem9 ==
  In1 : Inport
  Action Port : ActionPort  ActionType=else
  Fcn1 : Fcn  Expr=u(1)
  Fcn2 : Fcn  Expr=u(2)
  T1 : Outport
  T2 : Outport  Port=2
  wires:
  Fcn2/1 -> T2/1
  Fcn1/1 -> T1/1
  In1/1 -> Fcn2/1, Fcn1/1
